simulink model "HEV_SIMULATION"  (R2026a)
settings: Solver=VariableStepAuto  StopTime=20
undefined symbols (not defined in the file): air_density, Cd, frontal_area, vehicle_mass
settings Model: Creator=sai krishna  LastModifiedBy=sai krishna

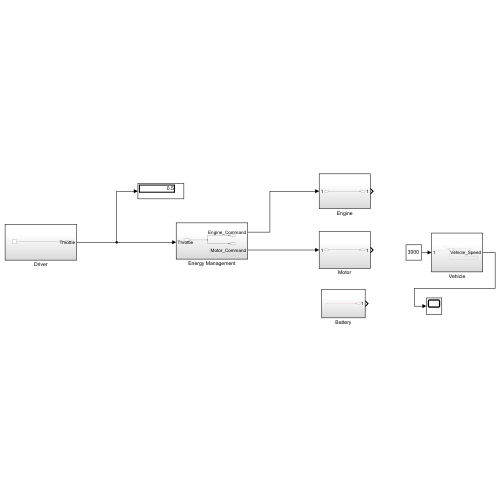
[thumbnail: Simulink's stored preview of the top-level diagram]
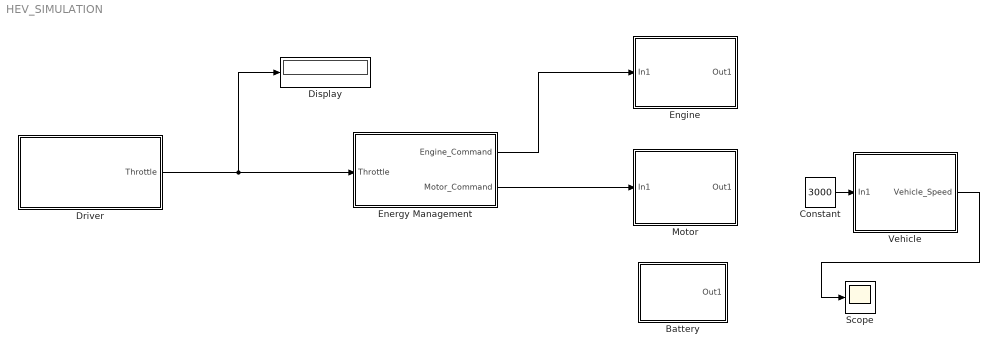
== system HEV_SIMULATION ==
  Battery : Subsystem
  Constant : Constant  Value=3000
  Display : Display
  Driver : Subsystem
  Energy Management : Subsystem
  Engine : Subsystem
  Motor : Subsystem
  Scope : Scope
      settings: ActiveDisplayYMinimum=-4.6685804279849759  ActiveDisplayYMaximum=42.017223851864792
  Vehicle : Subsystem
  wires:
  Driver/1(Throttle) -> Display/1, Energy Management/1(Throttle)
  Energy Management/1(Engine_Command) -> Engine/1(In1)
  Energy Management/2(Motor_Command) -> Motor/1(In1)
  Constant/1 -> Vehicle/1(In1)
  Vehicle/1(Vehicle_Speed) -> Scope/1

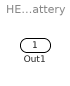
== system HEV_SIMULATION/Battery ==
  Out1 : Outport
  wires:
  ? -> Out1/1

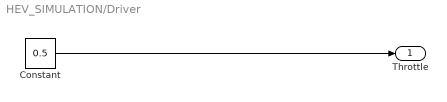
== system HEV_SIMULATION/Driver ==
  Constant : Constant  Value=0.5
  Throttle : Outport
  wires:
  Constant/1 -> Throttle/1

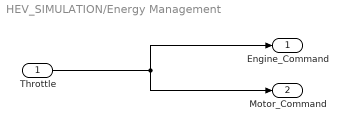
== system HEV_SIMULATION/Energy Management ==
  Throttle : Inport
  Engine_Command : Outport
  Motor_Command : Outport  Port=2
  wires:
  Throttle/1 -> Engine_Command/1, Motor_Command/1

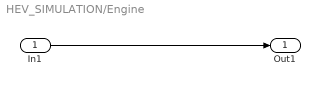
== system HEV_SIMULATION/Engine ==
  In1 : Inport
  Out1 : Outport
  wires:
  In1/1 -> Out1/1

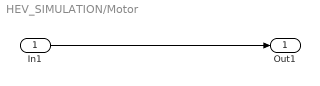
== system HEV_SIMULATION/Motor ==
  In1 : Inport
  Out1 : Outport
  wires:
  In1/1 -> Out1/1

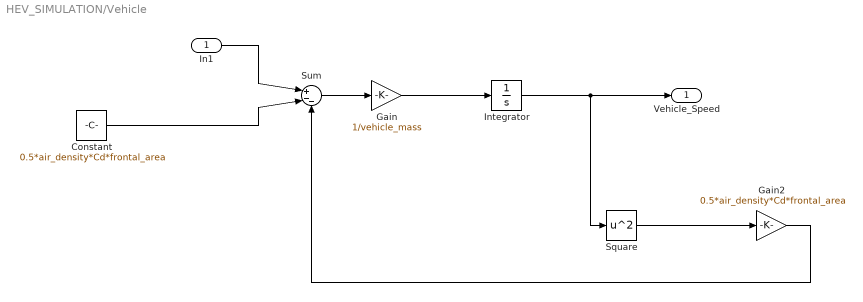
== system HEV_SIMULATION/Vehicle ==
  In1 : Inport
  Constant : Constant  Value=0.5*air_density*Cd*frontal_area
  Gain : Gain  Gain=1/vehicle_mass
  Gain2 : Gain  Gain=0.5*air_density*Cd*frontal_area
  Integrator : Integrator
  Square : Math  Operator=square
  Sum : Sum  Inputs=|+--
  Vehicle_Speed : Outport
  wires:
  Gain/1 -> Integrator/1
  Sum/1 -> Gain/1
  Integrator/1 -> Square/1, Vehicle_Speed/1
  In1/1 -> Sum/1
  Constant/1 -> Sum/2
  Square/1 -> Gain2/1
  Gain2/1 -> Sum/3
